simulink model "MotorSys"  (R2019a)
settings: Solver=VariableStepAuto  StartTime=0.0  StopTime=10.0  RelTol=1e-3
undefined symbols (not defined in the file or in its folder): DiscIntNeverNeededParam
libraries: simulink x2, fuzblock x2
settings Model: Creator=936305695  LastModifiedBy=936305695
settings SolverCC: AlgebraicLoopSolver=LineSearch

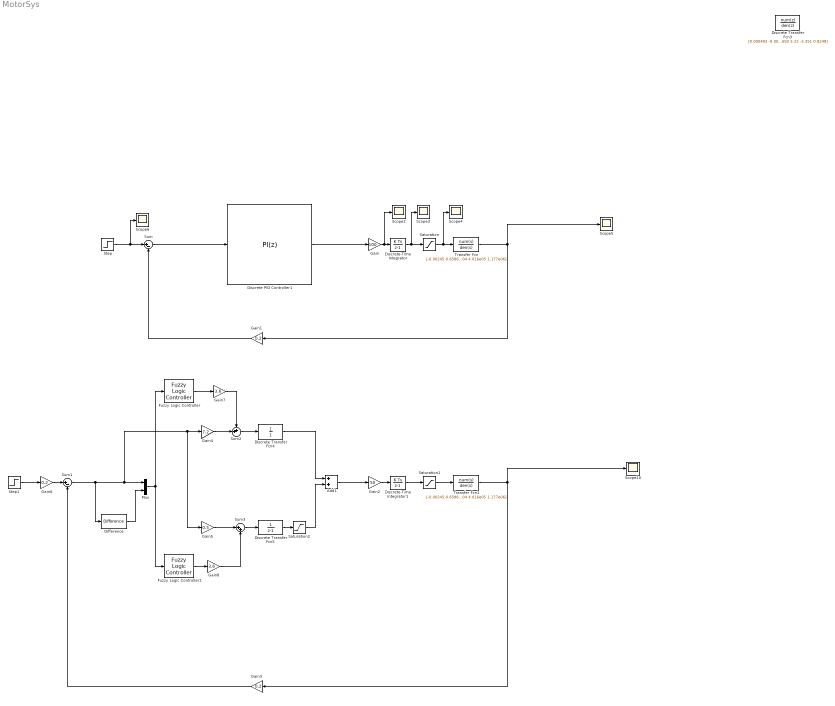
== system MotorSys ==
  Add1 : Sum
  Difference : simulink/Discrete/Difference  ICPrevInput=0.0  OutMin=[]  OutMax=[]  OutDataType=fixdt(1, 16)  OutScaling=2^-10  DoSatur=off
  Discrete Transfer Fcn3 : DiscreteTransferFcn  Numerator=[0.000493 -0.0006711 2.422e-05 0.0001617]  Denominator=[1 -3.693 5.22 -3.351 0.8248]  SampleTime=0.002
  Discrete Transfer Fcn4 : DiscreteTransferFcn  Denominator=[1]  SampleTime=0.002
  Discrete Transfer Fcn5 : DiscreteTransferFcn  Denominator=[1 -1]  SampleTime=0.002
  Discrete PID Controller1 : simulink/Continuous/PID Controller  Controller=PI  Form=Parallel  TimeDomain=Discrete-time  SampleTime=0.002  IntegratorMethod=Forward Euler  FilterMethod=Forward Euler  ControllerParametersSource=internal  P=3.6  I=0.2  D=0  UseFilter=off  N=100  TunerSelectOption=Transfer Function Based (PID Tuner App)  InitialConditionSource=internal  InitialConditionForIntegrator=0  InitialConditionForFilter=0  DifferentiatorICPrevScaledInput=0  ExternalReset=none  TrackingMode=off  Kt=1  LimitOutput=off  UpperSaturationLimit=inf  LowerSaturationLimit=-inf  LinearizeAsGain=off  AntiWindupMode=none  Kb=1  POutMin=[]  POutMax=[]  IOutMin=[]  IOutMax=[]  DOutMin=[]  DOutMax=[]  NOutMin=[]  NOutMax=[]  SumOutMin=[]  SumOutMax=[]  SaturationOutMin=[]  SaturationOutMax=[]  PParamMin=[]  PParamMax=[]  IParamMin=[]  IParamMax=[]  DParamMin=[]  DParamMax=[]  NParamMin=[]  NParamMax=[]  KbParamMin=[]  KbParamMax=[]  KtParamMin=[]  KtParamMax=[]  KbOutMin=[]  KbOutMax=[]  KtOutMin=[]  KtOutMax=[]  IntegratorOutMin=[]  IntegratorOutMax=[]  FilterOutMin=[]  FilterOutMax=[]  SumI1OutMin=[]  SumI1OutMax=[]  SumI2OutMin=[]  SumI2OutMax=[]  SumI3OutMin=[]  SumI3OutMax=[]  SumI4OutMin=[]  SumI4OutMax=[]  SumDOutMin=[]  SumDOutMax=[]  DifferentiatorOutMin=[]  DifferentiatorOutMax=[]  FilterDiffOutCoefMin=[]  FilterDiffOutCoefMax=[]  ReciprocalOutMin=[]  ReciprocalOutMax=[]  SumDenOutMin=[]  SumDenOutMax=[]  SumNumOutMin=[]  SumNumOutMax=[]  DivideOutMin=[]  DivideOutMax=[]  IntegratorContinuousStateAttributes=''  IntegratorStateMustResolveToSignalObject=off  IntegratorRTWStateStorageClass=Auto  FilterContinuousStateAttributes=''  FilterStateMustResolveToSignalObject=off  FilterRTWStateStorageClass=Auto  ParallelPVariant=InternalParameters  IdealPVariant=Disabled  IVariant=InternalParameters  DVariant=Disabled  IntegratorVariant=Discrete  SatVariant=Disabled  AWVariant=Passthrough  PCopyVariant=Disabled  TRVariant=Disabled  FdbkBlocksVariant=Forward  IdealPFdbkVariant=Disabled  SatFdbkVariant=Disabled  DerivativeFilterVariant=Disabled  NVariant=Disabled  NCopyVariant=Disabled_SignalSpec  FilterICVariant=Disabled  IntegratorICVariant=InternalICs  ExternalResetVariant=Disabled  TRSumVariant=Passthrough  SumFdbkVariant=Disabled  SumVariant=Sum_PI
  Discrete-Time Integrator : DiscreteIntegrator  SampleTime=0.002  ICPrevOutput=DiscIntNeverNeededParam  ICPrevScaledInput=DiscIntNeverNeededParam
  Discrete-Time Integrator1 : DiscreteIntegrator  SampleTime=0.002  ICPrevOutput=DiscIntNeverNeededParam  ICPrevScaledInput=DiscIntNeverNeededParam
  Fuzzy Logic Controller : fuzblock/Fuzzy Logic  Controller  FIS=mFuzzyKp  OutputSampleNumber=101  DataType=double  FuzzifiedInputs=off  RuleFiringStrengths=off  RuleOutputs=off  AggregatedOutputs=off  SimulateUsing=Interpreted execution  OutOfRangeInputValueMessage=warning  NoRuleFiredMessage=warning  EmptyOutputFuzzySetMessage=warning
  Fuzzy Logic Controller1 : fuzblock/Fuzzy Logic  Controller  FIS=mFuzzyKi  OutputSampleNumber=101  DataType=double  FuzzifiedInputs=off  RuleFiringStrengths=off  RuleOutputs=off  AggregatedOutputs=off  SimulateUsing=Interpreted execution  OutOfRangeInputValueMessage=warning  NoRuleFiredMessage=warning  EmptyOutputFuzzySetMessage=warning
  Gain : Gain  Gain=100
  Gain1 : Gain  Gain=0.2
  Gain2 : Gain  Gain=50
  Gain3 : Gain  Gain=0.2
  Gain4 : Gain  Gain=7.2
  Gain5 : Gain  Gain=0.5
  Gain6 : Gain  Gain=0.2
  Gain7 : Gain  Gain=3.6
  Gain8 : Gain  Gain=3.6
  Mux : Mux  Inputs=2
  Saturation : Saturate  UpperLimit=5000  LowerLimit=-5000
  Saturation1 : Saturate  UpperLimit=5000.0  LowerLimit=-5000.0
  Saturation2 : Saturate  UpperLimit=5.0  LowerLimit=-5.0
  Scope{2..6,10} (6 alike) : Scope
  Step : Step  Time=0.1  After=50  SampleTime=0.002
  Step1 : Step  Time=0  After=150.0  SampleTime=0.002
  Sum : Sum  Inputs=|+-
  Sum1 : Sum  Inputs=|+-
  Sum2 : Sum  Inputs=++|
  Sum3 : Sum  Inputs=|++
  Transfer Fcn : TransferFcn  Numerator=[-0.00245 0.6586 77.32 1.65e04 5.995e04]  Denominator=[1 63.17 2.603e04 4.016e05 1.177e06]
  Transfer Fcn1 : TransferFcn  Numerator=[-0.00245 0.6586 77.32 1.65e04 5.995e04]  Denominator=[1 63.17 2.603e04 4.016e05 1.177e06]
  wires:
  Discrete PID Controller1/1 -> Gain/1
  Transfer Fcn/1 -> Gain1/1, Scope5/1
  Step/1 -> Scope6/1, Sum/1
  Gain1/1 -> Sum/2
  Discrete-Time Integrator/1 -> Scope3/1, Saturation/1
  Gain/1 -> Scope2/1, Discrete-Time Integrator/1
  Saturation/1 -> Transfer Fcn/1, Scope4/1
  Saturation2/1 -> Add1/2
  Discrete Transfer Fcn5/1 -> Saturation2/1
  Add1/1 -> Gain2/1
  Discrete Transfer Fcn4/1 -> Add1/1
  Sum/1 -> Discrete PID Controller1/1
  Transfer Fcn1/1 -> Scope10/1, Gain3/1
  Saturation1/1 -> Transfer Fcn1/1
  Discrete-Time Integrator1/1 -> Saturation1/1
  Step1/1 -> Gain6/1
  Gain2/1 -> Discrete-Time Integrator1/1
  Gain3/1 -> Sum1/2
  Sum1/1 -> Difference/1, Gain5/1, Gain4/1, Mux/1
  Gain6/1 -> Sum1/1
  Gain4/1 -> Sum2/2
  Sum2/1 -> Discrete Transfer Fcn4/1
  Gain5/1 -> Sum3/1
  Sum3/1 -> Discrete Transfer Fcn5/1
  Mux/1 -> Fuzzy Logic Controller1/1, Fuzzy Logic Controller/1
  Difference/1 -> Mux/2
  Fuzzy Logic Controller/1 -> Gain7/1
  Gain7/1 -> Sum2/1
  Fuzzy Logic Controller1/1 -> Gain8/1
  Gain8/1 -> Sum3/2
